simulink model "PreviewCurvature"  (R2024a)
settings: configuration reference "csMultiInstance" (kept outside this file)
undefined symbols (not defined in the file or in its folder): LaneCurveParams_Max, LaneCurveParams_Min, PredictionTimeSteps, Ts
Description:
  | Software unit for preview curvature
settings Model: DataDictionary=DD_PreviewCurvature.sldd  EnableAccessToBaseWorkspace=off  Creator=The MathWorks, Inc.  LastModifiedBy=The MathWorks, Inc.
settings ConfigSetRef: SourceName=csMultiInstance

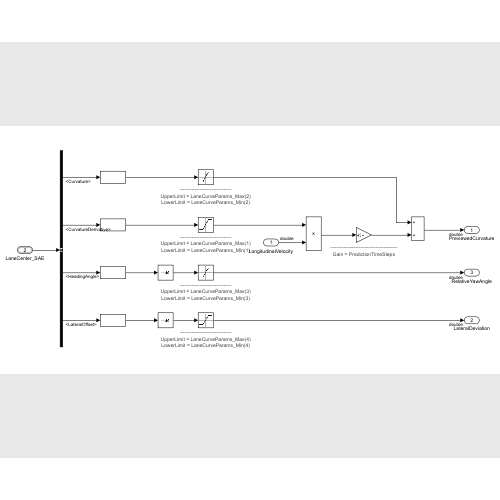
[thumbnail: Simulink's stored preview of the top-level diagram]
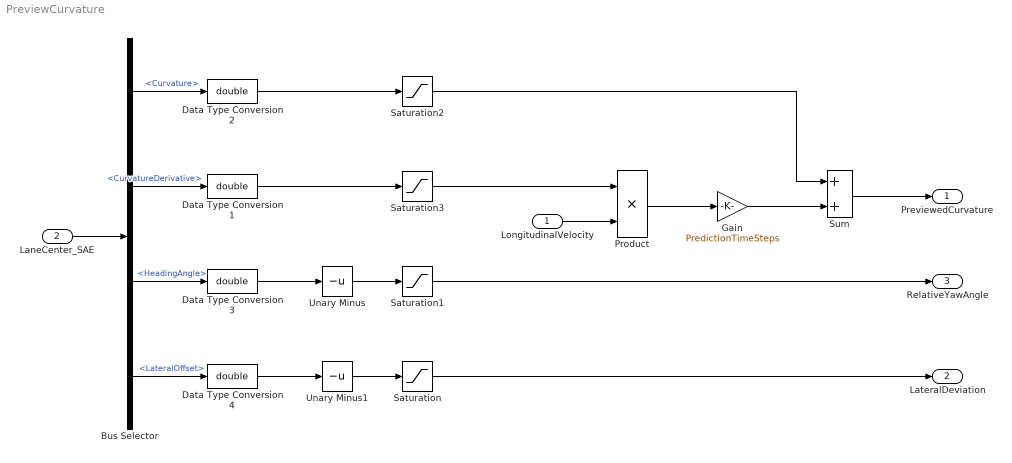
== system PreviewCurvature ==
  LongitudinalVelocity : Inport  OutDataTypeStr=double  Unit=m/s  PortDimensions=1  SampleTime=Ts
  LaneCenter_SAE : Inport  Port=2  OutDataTypeStr=Bus: BusLaneCenter  SampleTime=Ts
  Bus Selector : BusSelector  OutputSignals=Curvature,CurvatureDerivative,HeadingAngle,LateralOffset
  Data Type Conversion{1..4} (4 alike) : DataTypeConversion  OutDataTypeStr=double  SaturateOnIntegerOverflow=off  RndMeth=Floor
  Gain : Gain  Gain=PredictionTimeSteps
      settings: AttributesFormatString=|
      | ----------------------------------------
      | Gain = %<Gain>
  Product : Product
  Saturation : Saturate  UpperLimit=LaneCurveParams_Max(4)  LowerLimit=LaneCurveParams_Min(4)
      settings: AttributesFormatString=|
      | -------------------------------
      | UpperLimit = %<UpperLimit>
      | LowerLimit = %<LowerLimit>
  Saturation1 : Saturate  UpperLimit=LaneCurveParams_Max(3)  LowerLimit=LaneCurveParams_Min(3)
      settings: AttributesFormatString=|
      | -------------------------------
      | UpperLimit = %<UpperLimit>
      | LowerLimit = %<LowerLimit>
  Saturation2 : Saturate  UpperLimit=LaneCurveParams_Max(2)  LowerLimit=LaneCurveParams_Min(2)
      settings: AttributesFormatString=|
      | -------------------------------
      | UpperLimit = %<UpperLimit>
      | LowerLimit = %<LowerLimit>
  Saturation3 : Saturate  UpperLimit=LaneCurveParams_Max(1)  LowerLimit=LaneCurveParams_Min(1)
      settings: AttributesFormatString=|
      | -------------------------------
      | UpperLimit = %<UpperLimit>
      | LowerLimit = %<LowerLimit>
  Sum : Sum
  Unary Minus : UnaryMinus
  Unary Minus1 : UnaryMinus
  PreviewedCurvature : Outport  OutDataTypeStr=double  PortDimensions=PredictionNumSteps  VectorParamsAs1DForOutWhenUnconnected=off
  LateralDeviation : Outport  Port=2  OutDataTypeStr=double  VectorParamsAs1DForOutWhenUnconnected=off
  RelativeYawAngle : Outport  Port=3  OutDataTypeStr=double  VectorParamsAs1DForOutWhenUnconnected=off
  wires:
  Saturation1/1 -> RelativeYawAngle/1
  Saturation/1 -> LateralDeviation/1
  LaneCenter_SAE/1 -> Bus Selector/1
  Sum/1 -> PreviewedCurvature/1
  LongitudinalVelocity/1 -> Product/2
  Bus Selector/3 -> Data Type Conversion3/1  "<HeadingAngle>"
  Product/1 -> Gain/1
  Saturation3/1 -> Product/1
  Unary Minus/1 -> Saturation1/1
  Saturation2/1 -> Sum/1
  Data Type Conversion2/1 -> Saturation2/1
  Data Type Conversion3/1 -> Unary Minus/1
  Data Type Conversion4/1 -> Unary Minus1/1
  Gain/1 -> Sum/2
  Bus Selector/4 -> Data Type Conversion4/1  "<LateralOffset>"
  Data Type Conversion1/1 -> Saturation3/1
  Bus Selector/2 -> Data Type Conversion1/1  "<CurvatureDerivative>"
  Bus Selector/1 -> Data Type Conversion2/1  "<Curvature>"
  Unary Minus1/1 -> Saturation/1
